simulink model "Project_Model"  (R2022b)
settings: Solver=ode45  StartTime=0.0  StopTime=1000  MaxStep=1  RelTol=1e-7
values from neighbouring files (symbols this model uses):
  a = (Rp+Ra)/2    [trial_complete_project.m]    (also in trial_detumbling.m; trial_earth_pointing.m)
  A0 = Ax*Ay*Az    [trial_complete_project.m]    (also in trial_detumbling.m = [0.5391 0.1008 0.8362; -0.3591 0.9255 0.1200; -0.7618 -0.365; trial_earth_pointing.m = [-0.2505 -0.7848 0.5668; 0.7978 0.1644 0.5801; -0.5485 0.597)
  A1 = L1*L2    (= 0.06)    [trial_complete_project.m]    (also in trial_detumbling.m; trial_earth_pointing.m)
  A10 = A1    (= 0.06)    [trial_complete_project.m]    (also in trial_detumbling.m; trial_earth_pointing.m)
  A2 = A1    (= 0.06)    [trial_complete_project.m]    (also in trial_detumbling.m; trial_earth_pointing.m)
  A3 = L1*L3    (= 0.03)    [trial_complete_project.m]    (also in trial_detumbling.m; trial_earth_pointing.m)
  A4 = A3    (= 0.03)    [trial_complete_project.m]    (also in trial_detumbling.m; trial_earth_pointing.m)
  A5 = L2*L3    (= 0.02)    [trial_complete_project.m]    (also in trial_detumbling.m; trial_earth_pointing.m)
  A6 = A5    (= 0.02)    [trial_complete_project.m]    (also in trial_detumbling.m; trial_earth_pointing.m)
  A7 = A1    (= 0.06)    [trial_complete_project.m]    (also in trial_detumbling.m; trial_earth_pointing.m)
  A8 = A1    (= 0.06)    [trial_complete_project.m]    (also in trial_detumbling.m; trial_earth_pointing.m)
  A9 = A1    (= 0.06)    [trial_complete_project.m]    (also in trial_detumbling.m; trial_earth_pointing.m)
  a_s = 149600000    [trial_complete_project.m]    (also in trial_detumbling.m; trial_earth_pointing.m)
  alpha1 = 0.9    [trial_complete_project.m]    (also in trial_detumbling.m; trial_earth_pointing.m)
  alpha2 = 0.1    [trial_complete_project.m]    (also in trial_detumbling.m; trial_earth_pointing.m)
  alphaState_obs = -0.9    [trial_complete_project.m]    (also in trial_detumbling.m; trial_earth_pointing.m)
  an = (11.5*pi)/180    (= 0.200712863979)    [trial_complete_project.m]    (also in trial_detumbling.m; trial_earth_pointing.m)
  d = 0.05/2    (= 0.025)    [trial_complete_project.m]    (also in trial_detumbling.m; trial_earth_pointing.m)
  e = (Ra-Rp)/(Ra+Rp)    [trial_complete_project.m]    (also in trial_detumbling.m; trial_earth_pointing.m)
  e_s = 0.0167086    [trial_complete_project.m]    (also in trial_detumbling.m; trial_earth_pointing.m)
  g_vect = g_vect'.*1e-9    [trial_complete_project.m]    (also in trial_detumbling.m; trial_earth_pointing.m)
  gamma = 30*pi/180    (= 0.523598775598)    [trial_complete_project.m]    (also in trial_detumbling.m; trial_earth_pointing.m)
  h_vect = h_vect'.*1e-9    [trial_complete_project.m]    (also in trial_detumbling.m; trial_earth_pointing.m)
  i = 0*pi/180    (= 0)    [trial_complete_project.m]    (also in trial_detumbling.m; trial_earth_pointing.m)
  I_x = 0.059029338    [trial_complete_project.m]    (also in trial_detumbling.m; trial_earth_pointing.m = 0.093296)
  I_y = 0.116709338    [trial_complete_project.m]    (also in trial_detumbling.m; trial_earth_pointing.m = 0.161261916)
  I_z = 0.149968    [trial_complete_project.m]    (also in trial_detumbling.m; trial_earth_pointing.m = 0.160253916)
  kdx = kd*(I_x/I)    (= 1.44987726319)    [trial_complete_project.m]    (also in trial_detumbling.m; trial_earth_pointing.m = 2.6989394073)
  kdy = kd*(I_y/I)    (= 2.86661211697)    [trial_complete_project.m]    (also in trial_detumbling.m; trial_earth_pointing.m = 4.66511040119)
  kdz = kd*(I_z/I)    (= 3.68351061984)    [trial_complete_project.m]    (also in trial_detumbling.m; trial_earth_pointing.m = 4.63595019151)
  kpx = kp*(I_x/I)    (= 0.0163111192108)    [trial_complete_project.m]    (also in trial_detumbling.m; trial_earth_pointing.m = 0.0202420455548)
  kpy = kp*(I_y/I)    (= 0.0322493863159)    [trial_complete_project.m]    (also in trial_detumbling.m; trial_earth_pointing.m = 0.0349883280089)
  kpz = kp*(I_z/I)    (= 0.0414394944732)    [trial_complete_project.m]    (also in trial_detumbling.m; trial_earth_pointing.m = 0.0347696264363)
  kState_obs = 0.9    [trial_complete_project.m]    (also in trial_detumbling.m; trial_earth_pointing.m)
  L = 0.3/2    (= 0.15)    [trial_complete_project.m]    (also in trial_detumbling.m; trial_earth_pointing.m)
  m = [0.01 0.05 0.01]    [trial_complete_project.m]    (also in trial_detumbling.m; trial_earth_pointing.m)
  MIB = 5*1e-3    (= 0.005)    [trial_complete_project.m]    (also in trial_detumbling.m; trial_earth_pointing.m)
  mu = astroConstants(13)    [trial_complete_project.m]    (also in trial_detumbling.m; trial_earth_pointing.m)
  n = sqrt(mu/a^3)    [trial_complete_project.m]    (also in trial_detumbling.m; trial_earth_pointing.m)
  n_B = 13    [trial_complete_project.m]    (also in trial_detumbling.m; trial_earth_pointing.m)
  n_s = sqrt(mu_s/a_s^3)    [trial_complete_project.m]    (also in trial_detumbling.m; trial_earth_pointing.m)
  P = F_e/c    (= 4.52980041279e-06)    [trial_complete_project.m]    (also in trial_detumbling.m; trial_earth_pointing.m)
  P_E = F_earth/c    (= 2.23487943783e-06)    [trial_complete_project.m]    (also in trial_detumbling.m; trial_earth_pointing.m)
  pd_sc = 0.1    [trial_complete_project.m]    (also in trial_detumbling.m; trial_earth_pointing.m)
  pd_sp = 0.1    [trial_complete_project.m]    (also in trial_detumbling.m; trial_earth_pointing.m)
  ps_sc = 0.5    [trial_complete_project.m]    (also in trial_detumbling.m; trial_earth_pointing.m)
  ps_sp = 0.1    [trial_complete_project.m]    (also in trial_detumbling.m; trial_earth_pointing.m)
  r = astroConstants(23)    [trial_complete_project.m]    (also in trial_detumbling.m; trial_earth_pointing.m)
  r1 = [0;0;-L3/2] + c_m    [trial_complete_project.m]    (also in trial_detumbling.m; trial_earth_pointing.m)
  r10 = r9    [trial_complete_project.m]    (also in trial_detumbling.m; trial_earth_pointing.m)
  r2 = [0; 0 ;L3/2] + c_m    [trial_complete_project.m]    (also in trial_detumbling.m; trial_earth_pointing.m)
  r3 = [0; L2/2;0] + c_m    [trial_complete_project.m]    (also in trial_detumbling.m; trial_earth_pointing.m)
  r4 = [0; -L2/2;0] + c_m    [trial_complete_project.m]    (also in trial_detumbling.m; trial_earth_pointing.m)
  r5 = [-L1/2; 0 ;0] + c_m    [trial_complete_project.m]    (also in trial_detumbling.m; trial_earth_pointing.m)
  r6 = [L1/2; 0;0]+ c_m    [trial_complete_project.m]    (also in trial_detumbling.m; trial_earth_pointing.m)
  r7 = [-L1/2; 0 ; L3/2 + L1/2] + c_m    [trial_complete_project.m]    (also in trial_detumbling.m; trial_earth_pointing.m)
  r8 = r7    [trial_complete_project.m]    (also in trial_detumbling.m; trial_earth_pointing.m)
  r9 = [-L1/2; 0 ; -L3/2 - L1/2]    [trial_complete_project.m]    (also in trial_detumbling.m; trial_earth_pointing.m)
  RW = 0.002    [trial_complete_project.m]    (also in trial_detumbling.m; trial_earth_pointing.m)
  theta0 = 0    [trial_complete_project.m]    (also in trial_detumbling.m; trial_earth_pointing.m)
  Thruster_Power = 0.03    [trial_complete_project.m]    (also in trial_detumbling.m; trial_earth_pointing.m)
  w = [1 1 1 1]'    [trial_complete_project.m]    (also in trial_detumbling.m; trial_earth_pointing.m)
  w0_x = 1    [trial_complete_project.m]    (also in trial_detumbling.m; trial_earth_pointing.m = -0.008328)
  w0_y = 1    [trial_complete_project.m]    (also in trial_detumbling.m; trial_earth_pointing.m = 0.004962)
  w0_z = 1    [trial_complete_project.m]    (also in trial_detumbling.m; trial_earth_pointing.m = -0.0004756)
  w_E = (15.04*pi/180)/3600    (= 7.29159776389e-05)    [trial_complete_project.m]    (also in trial_detumbling.m; trial_earth_pointing.m)
libraries: matrix_library x28, vrlib x6, dspinverses x2
(part 3 of 3)

== system Project_Model/Environment/Magnetic Torque/MAGNETIC FIELD ==
  S/C position : Inport
  Clock : Clock
  Constant1 : Constant  Value=g_vect
  Constant2 : Constant  Value=h_vect
  MATLAB Function1 : MATLAB Function  TreatAsAtomicUnit=on
  MATLAB Function2 : MATLAB Function  TreatAsAtomicUnit=on
  "order n " : Constant  Value=n_B
  B_n : Outport
  wires:
  Constant2/1 -> MATLAB Function1/7(hS)
  Constant1/1 -> MATLAB Function1/6(gS)
  MATLAB Function2/3(lat) -> MATLAB Function1/4(lat)
  MATLAB Function2/4(lon) -> MATLAB Function1/5(lon)
  Clock/1 -> MATLAB Function2/2(t)
  MATLAB Function2/1(r) -> MATLAB Function1/2(r)
  S/C position/1 -> MATLAB Function2/1(R)
  MATLAB Function2/2(alpha) -> MATLAB Function1/3(alpha)
  "order n "/1 -> MATLAB Function1/1(n_B)
  MATLAB Function1/1(B) -> B_n/1  "B_n"

== system Project_Model/Environment/Magnetic Torque/Theta_integration ==
  Constant : Constant
  Constant1 : Constant  Value=e
  Constant2 : Constant  Value=e
  Constant3 : Constant
  Constant4 : Constant  Value=3/2
  Cos : Trigonometry  Operator=cos
  Divide : Product  Inputs=*/
  Gain : Gain  Gain=n
  Integrator : Integrator  InitialCondition=theta0
  Product : Product
  Scope : Scope
  Scope1 : Scope
  Square : Math  Operator=square
  Square1 : Math  Operator=square
  Square2 : Math  Operator=pow
  Sum : Sum  Inputs=|++
  Sum1 : Sum  Inputs=|+-
  Output : Outport
  wires:
  Constant1/1 -> Product/1
  Integrator/1 -> Output/1, Scope/1, Cos/1
  Constant3/1 -> Sum1/1
  Cos/1 -> Product/2
  Product/1 -> Sum/1
  Square1/1 -> Sum1/2
  Constant/1 -> Sum/2
  Sum1/1 -> Square2/1
  Constant2/1 -> Square1/1
  Square/1 -> Gain/1
  Divide/1 -> Scope1/1, Integrator/1
  Sum/1 -> Square/1
  Square2/1 -> Divide/2
  Constant4/1 -> Square2/2
  Gain/1 -> Divide/1

== system Project_Model/Environment/Magnetic Torque/r_N ==
  Input1 : Inport
  Constant : Constant  Value=i
  Constant2 : Constant
  Constant3 : Constant  Value=e
  Constant4 : Constant
  Constant5 : Constant  Value=e
  Cos : Trigonometry  Operator=cos
  Cos1 : Trigonometry  Operator=cos
  Cos4 : Trigonometry  Operator=cos
  Divide : Product  Inputs=*/  RndMeth=Zero  SaturateOnIntegerOverflow=on
  Gain : Gain  Gain=a
  Product{,1,4..5} (4 alike) : Product
  Sin : Trigonometry
  Sin1 : Trigonometry
  Square : Math  Operator=square
  Sum : Sum  Inputs=|+-
  Sum1 : Sum  Inputs=|++
  Vector Concatenate : Concatenate  NumInputs=3
  Output : Outport
  wires:
  Input1/1 -> Cos4/1, Cos/1, Sin/1
  Constant/1 -> Sin1/1, Cos1/1
  Cos/1 -> Vector Concatenate/1
  Sin/1 -> Product1/1, Product/1
  Cos1/1 -> Product/2
  Product/1 -> Vector Concatenate/2
  Sin1/1 -> Product1/2
  Product1/1 -> Vector Concatenate/3
  Constant4/1 -> Sum1/1
  Product5/1 -> Output/1
  Constant2/1 -> Sum/1
  Cos4/1 -> Product4/2
  Sum1/1 -> Divide/2
  Constant3/1 -> Square/1
  Product4/1 -> Sum1/2
  Square/1 -> Sum/2
  Gain/1 -> Divide/1
  Sum/1 -> Gain/1
  Constant5/1 -> Product4/1
  Divide/1 -> Product5/1
  Vector Concatenate/1 -> Product5/2

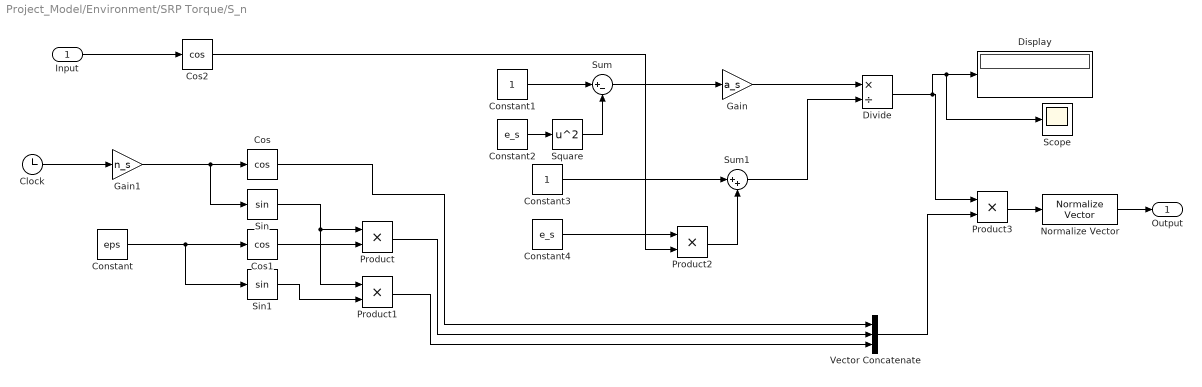
== system Project_Model/Environment/SRP Torque/S_n ==
  Input : Inport
  Clock : Clock
  Constant : Constant  Value=eps
  Constant1 : Constant
  Constant2 : Constant  Value=e_s
  Constant3 : Constant
  Constant4 : Constant  Value=e_s
  Cos : Trigonometry  Operator=cos
  Cos1 : Trigonometry  Operator=cos
  Cos2 : Trigonometry  Operator=cos
  Display : Display
  Divide : Product  Inputs=*/  RndMeth=Zero  SaturateOnIntegerOverflow=on
  Gain : Gain  Gain=a_s
  Gain1 : Gain  Gain=n_s
  Normalize Vector : vrlib/Utilities/Normalize Vector  maxzero=0
  Product{,1..3} (4 alike) : Product
  Scope : Scope
  Sin : Trigonometry
  Sin1 : Trigonometry
  Square : Math  Operator=square
  Sum : Sum  Inputs=|+-
  Sum1 : Sum  Inputs=|++
  Vector Concatenate : Concatenate  NumInputs=3
  Output : Outport
  wires:
  Product3/1 -> Normalize Vector/1
  Divide/1 -> Scope/1, Display/1, Product3/1
  Sum1/1 -> Divide/2
  Product2/1 -> Sum1/2
  Constant4/1 -> Product2/1
  Constant3/1 -> Sum1/1
  Gain/1 -> Divide/1
  Sum/1 -> Gain/1
  Square/1 -> Sum/2
  Constant2/1 -> Square/1
  Constant1/1 -> Sum/1
  Product1/1 -> Vector Concatenate/3
  Cos1/1 -> Product/2
  Sin1/1 -> Product1/2
  Constant/1 -> Cos1/1, Sin1/1
  Product/1 -> Vector Concatenate/2
  Cos/1 -> Vector Concatenate/1
  Sin/1 -> Product/1, Product1/1
  Vector Concatenate/1 -> Product3/2
  Clock/1 -> Gain1/1
  Gain1/1 -> Sin/1, Cos/1
  Input/1 -> Cos2/1
  Cos2/1 -> Product2/2
  Normalize Vector/1 -> Output/1

== system Project_Model/Environment/SRP Torque/Spacecraft Geometry ==
  Constant : Constant
  Gain : Gain  Gain=-1
  Gain1 : Gain  Gain=-1
  Gain2 : Gain  Gain=-1
  Vector Concatenate : Concatenate  NumInputs=3
  Vector Concatenate1 : Concatenate  NumInputs=3
  Vector Concatenate2 : Concatenate  NumInputs=3
  Zero : Constant  Value=0  OutDataTypeStr=Inherit: Inherit via back propagation
  Output : Outport
  Output1 : Outport  Port=2
  Output2 : Outport  Port=3
  Output3 : Outport  Port=4
  Output4 : Outport  Port=5
  Output5 : Outport  Port=6
  Output6 : Outport  Port=7
  Output7 : Outport  Port=8
  Output8 : Outport  Port=9
  Output9 : Outport  Port=10
  wires:
  Constant/1 -> Vector Concatenate2/3, Vector Concatenate/1, Vector Concatenate1/2
  Vector Concatenate1/1 -> Output3/1, Gain1/1
  Zero/1 -> Vector Concatenate2/2, Vector Concatenate2/1, Vector Concatenate1/3, Vector Concatenate/3, Vector Concatenate/2, Vector Concatenate1/1
  Vector Concatenate/1 -> Output8/1, Output6/1, Output4/1, Gain/1
  Vector Concatenate2/1 -> Gain2/1, Output/1
  Gain2/1 -> Output1/1
  Gain1/1 -> Output2/1
  Gain/1 -> Output9/1, Output7/1, Output5/1

== system Project_Model/Environment/SRP Torque/Subsystem ==
  Input : Inport
  Input1 : Inport  Port=2
  Constant : Constant
  Constant1 : Constant  Value=ps_sc
  Constant2 : Constant  Value=pd_sc
  Display : Display
  Dot Product : DotProduct  OutDataTypeStr=Inherit: Inherit via internal rule
  Gain : Gain  Gain=-P
  Gain1 : Gain  Gain=A1
  Gain2 : Gain  Gain=2
  Gain3 : Gain  Gain=2/3
  Product{,1..3} (4 alike) : Product
  Sum : Sum  Inputs=|+-
  Sum1 : Sum  Inputs=|++
  Sum2 : Sum  Inputs=|++
  Output : Outport
  Output1 : Outport  Port=2
  wires:
  Input1/1 -> Dot Product/2, Product3/2  "N_B"
  Product2/1 -> Sum2/1
  Product1/1 -> Sum1/1
  Constant2/1 -> Gain3/1
  Sum/1 -> Product1/1
  Constant1/1 -> Gain2/1, Sum/2
  Sum1/1 -> Product/2
  Product/1 -> Display/1, Output/1
  Dot Product/1 -> Output1/1, Product2/2, Gain/1
  Gain/1 -> Gain1/1
  Gain1/1 -> Product/1
  Sum2/1 -> Product3/1
  Input/1 -> Product1/2, Dot Product/1  "S-B"
  Gain2/1 -> Product2/1
  Constant/1 -> Sum/1
  Product3/1 -> Sum1/2
  Gain3/1 -> Sum2/2

== system Project_Model/Environment/SRP Torque/Subsystem10 ==
  Input : Inport
  Input1 : Inport  Port=2
  Constant : Constant
  Constant1 : Constant  Value=ps_sp
  Constant2 : Constant  Value=pd_sp
  Dot Product : DotProduct  OutDataTypeStr=Inherit: Inherit via internal rule
  Gain : Gain  Gain=-P
  Gain1 : Gain  Gain=A10
  Gain2 : Gain  Gain=2
  Gain3 : Gain  Gain=2/3
  Product{,1..3} (4 alike) : Product
  Sum : Sum  Inputs=|+-
  Sum1 : Sum  Inputs=|++
  Sum2 : Sum  Inputs=|++
  Output : Outport
  Output1 : Outport  Port=2
  wires:
  Gain3/1 -> Sum2/2
  Product3/1 -> Sum1/2
  Constant/1 -> Sum/1
  Gain2/1 -> Product2/1
  Input/1 -> Dot Product/1, Product1/2  "S-B"
  Sum2/1 -> Product3/1
  Gain1/1 -> Product/1
  Gain/1 -> Gain1/1
  Dot Product/1 -> Gain/1, Product2/2, Output1/1
  Product/1 -> Output/1
  Sum1/1 -> Product/2
  Constant1/1 -> Sum/2, Gain2/1
  Sum/1 -> Product1/1
  Constant2/1 -> Gain3/1
  Product1/1 -> Sum1/1
  Product2/1 -> Sum2/1
  Input1/1 -> Product3/2, Dot Product/2  "N_B"

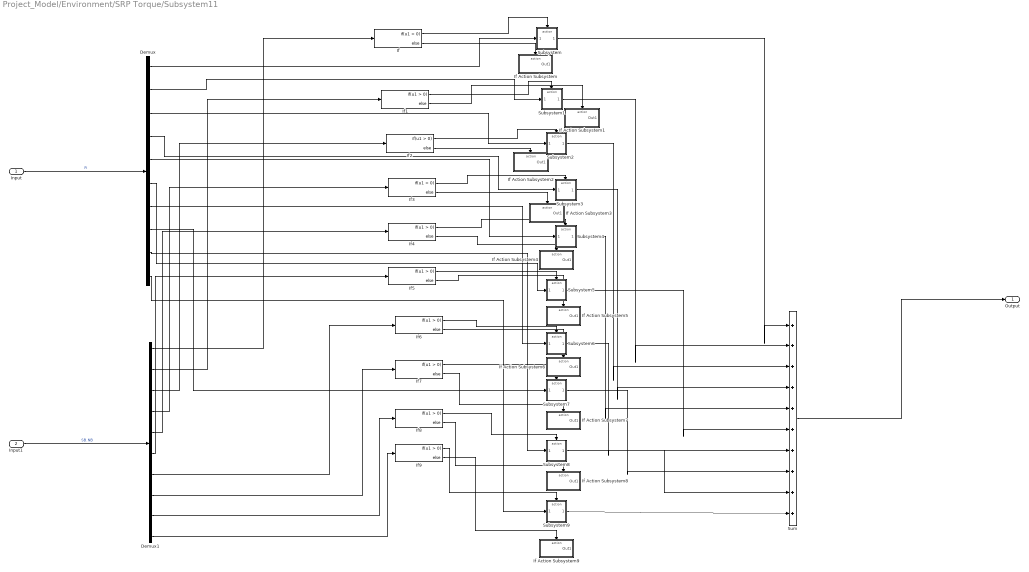
== system Project_Model/Environment/SRP Torque/Subsystem11 ==
  Input : Inport
  Input1 : Inport  Port=2
  Demux : Demux  Outputs=10
  Demux1 : Demux  Outputs=10
  If{,1..9} (10 alike) : If  ZeroCross=off
  If Action Subsystem : Subsystem  TreatAsAtomicUnit=on
  If Action Subsystem1 : Subsystem  TreatAsAtomicUnit=on
  If Action Subsystem2 : Subsystem  TreatAsAtomicUnit=on
  If Action Subsystem3 : Subsystem  TreatAsAtomicUnit=on
  If Action Subsystem4 : Subsystem  TreatAsAtomicUnit=on
  If Action Subsystem5 : Subsystem  TreatAsAtomicUnit=on
  If Action Subsystem6 : Subsystem  TreatAsAtomicUnit=on
  If Action Subsystem7 : Subsystem  TreatAsAtomicUnit=on
  If Action Subsystem8 : Subsystem  TreatAsAtomicUnit=on
  If Action Subsystem9 : Subsystem  TreatAsAtomicUnit=on
  Subsystem : Subsystem
  Subsystem1 : Subsystem
  Subsystem2 : Subsystem
  Subsystem3 : Subsystem
  Subsystem4 : Subsystem
  Subsystem5 : Subsystem
  Subsystem6 : Subsystem
  Subsystem7 : Subsystem
  Subsystem8 : Subsystem
  Subsystem9 : Subsystem
  Sum : Sum  Inputs=|++++++++++
  Output : Outport
  wires:
  Input/1 -> Demux/1  "Fi"
  Input1/1 -> Demux1/1  "SB.NB"
  Demux1/1 -> If/1
  Demux/1 -> Subsystem/1(Input3)
  Demux1/2 -> If1/1
  Demux1/3 -> If2/1
  Demux1/4 -> If3/1
  Demux1/5 -> If4/1
  Demux1/6 -> If5/1
  Demux1/7 -> If6/1
  Demux1/8 -> If7/1
  Demux1/9 -> If8/1
  Demux1/10 -> If9/1
  Demux/2 -> Subsystem1/1(Input3)
  Demux/3 -> Subsystem2/1(Input3)
  Demux/4 -> Subsystem3/1(Input3)
  Demux/5 -> Subsystem4/1(Input3)
  Demux/6 -> Subsystem5/1(Input3)
  Demux/7 -> Subsystem6/1(Input3)
  Demux/8 -> Subsystem7/1(Input3)
  Demux/9 -> Subsystem8/1(Input3)
  Demux/10 -> Subsystem9/1(Input3)
  Subsystem/1(Output) -> Sum/1
  Subsystem1/1(Output) -> Sum/2
  Subsystem2/1(Output) -> Sum/3
  Subsystem3/1(Output) -> Sum/4
  Subsystem4/1(Output) -> Sum/5
  Subsystem5/1(Output) -> Sum/6
  Subsystem6/1(Output) -> Sum/7
  Subsystem7/1(Output) -> Sum/8
  Subsystem8/1(Output) -> Sum/9
  Subsystem9/1(Output) -> Sum/10
  If/1 -> Subsystem/Action
  If/2 -> If Action Subsystem/Action
  If1/1 -> Subsystem1/Action
  If1/2 -> If Action Subsystem1/Action
  If2/2 -> If Action Subsystem2/Action
  If2/1 -> Subsystem2/Action
  If3/2 -> If Action Subsystem3/Action
  If3/1 -> Subsystem3/Action
  If4/2 -> If Action Subsystem4/Action
  If4/1 -> Subsystem4/Action
  If5/2 -> If Action Subsystem5/Action
  If5/1 -> Subsystem5/Action
  If6/2 -> If Action Subsystem6/Action
  If6/1 -> Subsystem6/Action
  If7/2 -> If Action Subsystem7/Action
  If7/1 -> Subsystem7/Action
  If8/2 -> If Action Subsystem8/Action
  If8/1 -> Subsystem8/Action
  If9/2 -> If Action Subsystem9/Action
  If9/1 -> Subsystem9/Action
  Sum/1 -> Output/1

== system Project_Model/Environment/SRP Torque/Subsystem2 ==
  Input : Inport
  Input1 : Inport  Port=2
  Constant : Constant
  Constant1 : Constant  Value=ps_sc
  Constant2 : Constant  Value=pd_sc
  Dot Product : DotProduct  OutDataTypeStr=Inherit: Inherit via internal rule
  Gain : Gain  Gain=-P
  Gain1 : Gain  Gain=A2
  Gain2 : Gain  Gain=2
  Gain3 : Gain  Gain=2/3
  Product{,1..3} (4 alike) : Product
  Sum : Sum  Inputs=|+-
  Sum1 : Sum  Inputs=|++
  Sum2 : Sum  Inputs=|++
  Output : Outport
  Output1 : Outport  Port=2
  wires:
  Gain3/1 -> Sum2/2
  Product3/1 -> Sum1/2
  Constant/1 -> Sum/1
  Gain2/1 -> Product2/1
  Input/1 -> Dot Product/1, Product1/2  "S-B"
  Sum2/1 -> Product3/1
  Gain1/1 -> Product/1
  Gain/1 -> Gain1/1
  Dot Product/1 -> Gain/1, Product2/2, Output1/1
  Product/1 -> Output/1
  Sum1/1 -> Product/2
  Constant1/1 -> Sum/2, Gain2/1
  Sum/1 -> Product1/1
  Constant2/1 -> Gain3/1
  Product1/1 -> Sum1/1
  Product2/1 -> Sum2/1
  Input1/1 -> Product3/2, Dot Product/2  "N_B"

== system Project_Model/Environment/SRP Torque/Subsystem3 ==
  Input : Inport
  Input1 : Inport  Port=2
  Constant : Constant
  Constant1 : Constant  Value=ps_sc
  Constant2 : Constant  Value=pd_sc
  Dot Product : DotProduct  OutDataTypeStr=Inherit: Inherit via internal rule
  Gain : Gain  Gain=-P
  Gain1 : Gain  Gain=A3
  Gain2 : Gain  Gain=2
  Gain3 : Gain  Gain=2/3
  Product{,1..3} (4 alike) : Product
  Sum : Sum  Inputs=|+-
  Sum1 : Sum  Inputs=|++
  Sum2 : Sum  Inputs=|++
  Output : Outport
  Output1 : Outport  Port=2
  wires:
  Input1/1 -> Dot Product/2, Product3/2  "N_B"
  Product2/1 -> Sum2/1
  Product1/1 -> Sum1/1
  Constant2/1 -> Gain3/1
  Sum/1 -> Product1/1
  Constant1/1 -> Gain2/1, Sum/2
  Sum1/1 -> Product/2
  Product/1 -> Output/1
  Dot Product/1 -> Output1/1, Product2/2, Gain/1
  Gain/1 -> Gain1/1
  Gain1/1 -> Product/1
  Sum2/1 -> Product3/1
  Input/1 -> Product1/2, Dot Product/1  "S-B"
  Gain2/1 -> Product2/1
  Constant/1 -> Sum/1
  Product3/1 -> Sum1/2
  Gain3/1 -> Sum2/2

== system Project_Model/Environment/SRP Torque/Subsystem4 ==
  Input : Inport
  Input1 : Inport  Port=2
  Constant : Constant
  Constant1 : Constant  Value=ps_sc
  Constant2 : Constant  Value=pd_sc
  Dot Product : DotProduct  OutDataTypeStr=Inherit: Inherit via internal rule
  Gain : Gain  Gain=-P
  Gain1 : Gain  Gain=A4
  Gain2 : Gain  Gain=2
  Gain3 : Gain  Gain=2/3
  Product{,1..3} (4 alike) : Product
  Sum : Sum  Inputs=|+-
  Sum1 : Sum  Inputs=|++
  Sum2 : Sum  Inputs=|++
  Output : Outport
  Output1 : Outport  Port=2
  wires:
  Gain3/1 -> Sum2/2
  Product3/1 -> Sum1/2
  Constant/1 -> Sum/1
  Gain2/1 -> Product2/1
  Input/1 -> Dot Product/1, Product1/2  "S-B"
  Sum2/1 -> Product3/1
  Gain1/1 -> Product/1
  Gain/1 -> Gain1/1
  Dot Product/1 -> Gain/1, Product2/2, Output1/1
  Product/1 -> Output/1
  Sum1/1 -> Product/2
  Constant1/1 -> Sum/2, Gain2/1
  Sum/1 -> Product1/1
  Constant2/1 -> Gain3/1
  Product1/1 -> Sum1/1
  Product2/1 -> Sum2/1
  Input1/1 -> Product3/2, Dot Product/2  "N_B"

== system Project_Model/Environment/SRP Torque/Subsystem5 ==
  Input : Inport
  Input1 : Inport  Port=2
  Constant : Constant
  Constant1 : Constant  Value=ps_sc
  Constant2 : Constant  Value=pd_sc
  Dot Product : DotProduct  OutDataTypeStr=Inherit: Inherit via internal rule
  Gain : Gain  Gain=-P
  Gain1 : Gain  Gain=A5
  Gain2 : Gain  Gain=2
  Gain3 : Gain  Gain=2/3
  Product{,1..3} (4 alike) : Product
  Sum : Sum  Inputs=|+-
  Sum1 : Sum  Inputs=|++
  Sum2 : Sum  Inputs=|++
  Output : Outport
  Output1 : Outport  Port=2
  wires:
  Input1/1 -> Dot Product/2, Product3/2  "N_B"
  Product2/1 -> Sum2/1
  Product1/1 -> Sum1/1
  Constant2/1 -> Gain3/1
  Sum/1 -> Product1/1
  Constant1/1 -> Gain2/1, Sum/2
  Sum1/1 -> Product/2
  Product/1 -> Output/1
  Dot Product/1 -> Output1/1, Product2/2, Gain/1
  Gain/1 -> Gain1/1
  Gain1/1 -> Product/1
  Sum2/1 -> Product3/1
  Input/1 -> Product1/2, Dot Product/1  "S-B"
  Gain2/1 -> Product2/1
  Constant/1 -> Sum/1
  Product3/1 -> Sum1/2
  Gain3/1 -> Sum2/2

== system Project_Model/Environment/SRP Torque/Subsystem6 ==
  Input : Inport
  Input1 : Inport  Port=2
  Constant : Constant
  Constant1 : Constant  Value=ps_sc
  Constant2 : Constant  Value=pd_sc
  Dot Product : DotProduct  OutDataTypeStr=Inherit: Inherit via internal rule
  Gain : Gain  Gain=-P
  Gain1 : Gain  Gain=A6
  Gain2 : Gain  Gain=2
  Gain3 : Gain  Gain=2/3
  Product{,1..3} (4 alike) : Product
  Sum : Sum  Inputs=|+-
  Sum1 : Sum  Inputs=|++
  Sum2 : Sum  Inputs=|++
  Output : Outport
  Output1 : Outport  Port=2
  wires:
  Gain3/1 -> Sum2/2
  Product3/1 -> Sum1/2
  Constant/1 -> Sum/1
  Gain2/1 -> Product2/1
  Input/1 -> Dot Product/1, Product1/2  "S-B"
  Sum2/1 -> Product3/1
  Gain1/1 -> Product/1
  Gain/1 -> Gain1/1
  Dot Product/1 -> Gain/1, Product2/2, Output1/1
  Product/1 -> Output/1
  Sum1/1 -> Product/2
  Constant1/1 -> Sum/2, Gain2/1
  Sum/1 -> Product1/1
  Constant2/1 -> Gain3/1
  Product1/1 -> Sum1/1
  Product2/1 -> Sum2/1
  Input1/1 -> Product3/2, Dot Product/2  "N_B"

== system Project_Model/Environment/SRP Torque/Subsystem7 ==
  Input : Inport
  Input1 : Inport  Port=2
  Constant : Constant
  Constant1 : Constant  Value=ps_sp
  Constant2 : Constant  Value=pd_sp
  Dot Product : DotProduct  OutDataTypeStr=Inherit: Inherit via internal rule
  Gain : Gain  Gain=-P
  Gain1 : Gain  Gain=A7
  Gain2 : Gain  Gain=2
  Gain3 : Gain  Gain=2/3
  Product{,1..3} (4 alike) : Product
  Sum : Sum  Inputs=|+-
  Sum1 : Sum  Inputs=|++
  Sum2 : Sum  Inputs=|++
  Output : Outport
  Output1 : Outport  Port=2
  wires:
  Input1/1 -> Dot Product/2, Product3/2  "N_B"
  Product2/1 -> Sum2/1
  Product1/1 -> Sum1/1
  Constant2/1 -> Gain3/1
  Sum/1 -> Product1/1
  Constant1/1 -> Gain2/1, Sum/2
  Sum1/1 -> Product/2
  Product/1 -> Output/1
  Dot Product/1 -> Output1/1, Product2/2, Gain/1
  Gain/1 -> Gain1/1
  Gain1/1 -> Product/1
  Sum2/1 -> Product3/1
  Input/1 -> Product1/2, Dot Product/1  "S-B"
  Gain2/1 -> Product2/1
  Constant/1 -> Sum/1
  Product3/1 -> Sum1/2
  Gain3/1 -> Sum2/2

== system Project_Model/Environment/SRP Torque/Subsystem8 ==
  Input : Inport
  Input1 : Inport  Port=2
  Constant : Constant
  Constant1 : Constant  Value=ps_sp
  Constant2 : Constant  Value=pd_sp
  Dot Product : DotProduct  OutDataTypeStr=Inherit: Inherit via internal rule
  Gain : Gain  Gain=-P
  Gain1 : Gain  Gain=A8
  Gain2 : Gain  Gain=2
  Gain3 : Gain  Gain=2/3
  Product{,1..3} (4 alike) : Product
  Sum : Sum  Inputs=|+-
  Sum1 : Sum  Inputs=|++
  Sum2 : Sum  Inputs=|++
  Output : Outport
  Output1 : Outport  Port=2
  wires:
  Gain3/1 -> Sum2/2
  Product3/1 -> Sum1/2
  Constant/1 -> Sum/1
  Gain2/1 -> Product2/1
  Input/1 -> Dot Product/1, Product1/2  "S-B"
  Sum2/1 -> Product3/1
  Gain1/1 -> Product/1
  Gain/1 -> Gain1/1
  Dot Product/1 -> Gain/1, Product2/2, Output1/1
  Product/1 -> Output/1
  Sum1/1 -> Product/2
  Constant1/1 -> Sum/2, Gain2/1
  Sum/1 -> Product1/1
  Constant2/1 -> Gain3/1
  Product1/1 -> Sum1/1
  Product2/1 -> Sum2/1
  Input1/1 -> Product3/2, Dot Product/2  "N_B"

== system Project_Model/Environment/SRP Torque/Subsystem9 ==
  Input : Inport
  Input1 : Inport  Port=2
  Constant : Constant
  Constant1 : Constant  Value=ps_sp
  Constant2 : Constant  Value=pd_sp
  Dot Product : DotProduct  OutDataTypeStr=Inherit: Inherit via internal rule
  Gain : Gain  Gain=-P
  Gain1 : Gain  Gain=A9
  Gain2 : Gain  Gain=2
  Gain3 : Gain  Gain=2/3
  Product{,1..3} (4 alike) : Product
  Sum : Sum  Inputs=|+-
  Sum1 : Sum  Inputs=|++
  Sum2 : Sum  Inputs=|++
  Output : Outport
  Output1 : Outport  Port=2
  wires:
  Input1/1 -> Dot Product/2, Product3/2  "N_B"
  Product2/1 -> Sum2/1
  Product1/1 -> Sum1/1
  Constant2/1 -> Gain3/1
  Sum/1 -> Product1/1
  Constant1/1 -> Gain2/1, Sum/2
  Sum1/1 -> Product/2
  Product/1 -> Output/1
  Dot Product/1 -> Output1/1, Product2/2, Gain/1
  Gain/1 -> Gain1/1
  Gain1/1 -> Product/1
  Sum2/1 -> Product3/1
  Input/1 -> Product1/2, Dot Product/1  "S-B"
  Gain2/1 -> Product2/1
  Constant/1 -> Sum/1
  Product3/1 -> Sum1/2
  Gain3/1 -> Sum2/2

== system Project_Model/Environment/SRP Torque/Theta_integration ==
  Constant : Constant
  Constant1 : Constant  Value=e
  Constant2 : Constant  Value=e
  Constant3 : Constant
  Constant4 : Constant  Value=3/2
  Cos : Trigonometry  Operator=cos
  Divide : Product  Inputs=*/
  Gain : Gain  Gain=n
  Integrator : Integrator  InitialCondition=theta0
  Product : Product
  Scope : Scope
  Square : Math  Operator=square
  Square1 : Math  Operator=square
  Square2 : Math  Operator=pow
  Sum : Sum  Inputs=|++
  Sum1 : Sum  Inputs=|+-
  Output : Outport
  wires:
  Gain/1 -> Divide/1
  Constant4/1 -> Square2/2
  Square2/1 -> Divide/2
  Sum/1 -> Square/1
  Divide/1 -> Integrator/1
  Square/1 -> Gain/1
  Constant2/1 -> Square1/1
  Sum1/1 -> Square2/1
  Constant/1 -> Sum/2
  Square1/1 -> Sum1/2
  Product/1 -> Sum/1
  Cos/1 -> Product/2
  Constant3/1 -> Sum1/1
  Integrator/1 -> Cos/1, Scope/1, Output/1
  Constant1/1 -> Product/1

== system Project_Model/Reaction Wheel/If Action Subsystem/If Action Subsystem ==
  Action Port : ActionPort  ActionPortLabel=if(u1 <RWmin)
  Constant : Constant  Value=0
  Out1 : Outport
  wires:
  Constant/1 -> Out1/1

== system Project_Model/Reaction Wheel/If Action Subsystem/If Action Subsystem1 ==
  Action Port : ActionPort  ActionPortLabel=elseif(u1>=RW)
  Constant : Constant  Value=RW
  Out1 : Outport
  wires:
  Constant/1 -> Out1/1

== system Project_Model/Reaction Wheel/If Action Subsystem/If Action Subsystem2 ==
  Input : Inport
  Action Port : ActionPort  ActionPortLabel=else
  Out1 : Outport
  wires:
  Input/1 -> Out1/1

== system Project_Model/Reaction Wheel/If Action Subsystem1/If Action Subsystem ==
  Action Port : ActionPort  ActionPortLabel=if(u1 >-RWmin)
  Constant : Constant  Value=0
  Out1 : Outport
  wires:
  Constant/1 -> Out1/1

== system Project_Model/Reaction Wheel/If Action Subsystem1/If Action Subsystem1 ==
  Action Port : ActionPort  ActionPortLabel=elseif(u1<=-RW)
  Constant : Constant  Value=-RW
  Out1 : Outport
  wires:
  Constant/1 -> Out1/1

== system Project_Model/Reaction Wheel/If Action Subsystem1/If Action Subsystem2 ==
  Input : Inport
  Action Port : ActionPort  ActionPortLabel=else
  Out1 : Outport
  wires:
  Input/1 -> Out1/1

== system Project_Model/Reaction Wheel/If Action Subsystem2/If Action Subsystem ==
  Action Port : ActionPort  ActionPortLabel=if(u1 <RWmin)
  Constant : Constant  Value=0
  Out1 : Outport
  wires:
  Constant/1 -> Out1/1

== system Project_Model/Reaction Wheel/If Action Subsystem2/If Action Subsystem1 ==
  Action Port : ActionPort  ActionPortLabel=elseif(u1>=RW)
  Constant : Constant  Value=RW
  Out1 : Outport
  wires:
  Constant/1 -> Out1/1

== system Project_Model/Reaction Wheel/If Action Subsystem2/If Action Subsystem2 ==
  Input : Inport
  Action Port : ActionPort  ActionPortLabel=else
  Out1 : Outport
  wires:
  Input/1 -> Out1/1

== system Project_Model/Reaction Wheel/If Action Subsystem3/If Action Subsystem ==
  Action Port : ActionPort  ActionPortLabel=if(u1 >-RWmin)
  Constant : Constant  Value=0
  Out1 : Outport
  wires:
  Constant/1 -> Out1/1

== system Project_Model/Reaction Wheel/If Action Subsystem3/If Action Subsystem1 ==
  Action Port : ActionPort  ActionPortLabel=elseif(u1<=-RW)
  Constant : Constant  Value=-RW
  Out1 : Outport
  wires:
  Constant/1 -> Out1/1

== system Project_Model/Reaction Wheel/If Action Subsystem3/If Action Subsystem2 ==
  Input : Inport
  Action Port : ActionPort  ActionPortLabel=else
  Out1 : Outport
  wires:
  Input/1 -> Out1/1

== system Project_Model/Reaction Wheel/If Action Subsystem4/If Action Subsystem ==
  Action Port : ActionPort  ActionPortLabel=if(u1 <RWmin)
  Constant : Constant  Value=0
  Out1 : Outport
  wires:
  Constant/1 -> Out1/1

== system Project_Model/Reaction Wheel/If Action Subsystem4/If Action Subsystem1 ==
  Action Port : ActionPort  ActionPortLabel=elseif(u1>=RW)
  Constant : Constant  Value=RW
  Out1 : Outport
  wires:
  Constant/1 -> Out1/1

== system Project_Model/Reaction Wheel/If Action Subsystem4/If Action Subsystem2 ==
  Input : Inport
  Action Port : ActionPort  ActionPortLabel=else
  Out1 : Outport
  wires:
  Input/1 -> Out1/1

== system Project_Model/Reaction Wheel/If Action Subsystem5/If Action Subsystem ==
  Action Port : ActionPort  ActionPortLabel=if(u1 >-RWmin)
  Constant : Constant  Value=0
  Out1 : Outport
  wires:
  Constant/1 -> Out1/1

== system Project_Model/Reaction Wheel/If Action Subsystem5/If Action Subsystem1 ==
  Action Port : ActionPort  ActionPortLabel=elseif(u1<=-RW)
  Constant : Constant  Value=-RW
  Out1 : Outport
  wires:
  Constant/1 -> Out1/1

== system Project_Model/Reaction Wheel/If Action Subsystem5/If Action Subsystem2 ==
  Input : Inport
  Action Port : ActionPort  ActionPortLabel=else
  Out1 : Outport
  wires:
  Input/1 -> Out1/1

== system Project_Model/Environment/ERP Torque/Subsystem11/If Action Subsystem ==
  Action Port : ActionPort  ActionPortLabel=else
  Constant : Constant  Value=[0 0 0]'
  Out1 : Outport
  wires:
  Constant/1 -> Out1/1

== system Project_Model/Environment/ERP Torque/Subsystem11/If Action Subsystem1 ==
  Action Port : ActionPort  ActionPortLabel=else
  Constant : Constant  Value=[0 0 0]'
  Out1 : Outport
  wires:
  Constant/1 -> Out1/1

== system Project_Model/Environment/ERP Torque/Subsystem11/If Action Subsystem2 ==
  Action Port : ActionPort  ActionPortLabel=else
  Constant : Constant  Value=[0 0 0]'
  Out1 : Outport
  wires:
  Constant/1 -> Out1/1

== system Project_Model/Environment/ERP Torque/Subsystem11/If Action Subsystem3 ==
  Action Port : ActionPort  ActionPortLabel=else
  Constant : Constant  Value=[0 0 0]'
  Out1 : Outport
  wires:
  Constant/1 -> Out1/1

== system Project_Model/Environment/ERP Torque/Subsystem11/If Action Subsystem4 ==
  Action Port : ActionPort  ActionPortLabel=else
  Constant : Constant  Value=[0 0 0]'
  Out1 : Outport
  wires:
  Constant/1 -> Out1/1

== system Project_Model/Environment/ERP Torque/Subsystem11/If Action Subsystem5 ==
  Action Port : ActionPort  ActionPortLabel=else
  Constant : Constant  Value=[0 0 0]'
  Out1 : Outport
  wires:
  Constant/1 -> Out1/1

== system Project_Model/Environment/ERP Torque/Subsystem11/If Action Subsystem6 ==
  Action Port : ActionPort  ActionPortLabel=else
  Constant : Constant  Value=[0 0 0]'
  Out1 : Outport
  wires:
  Constant/1 -> Out1/1

== system Project_Model/Environment/ERP Torque/Subsystem11/If Action Subsystem7 ==
  Action Port : ActionPort  ActionPortLabel=else
  Constant : Constant  Value=[0 0 0]'
  Out1 : Outport
  wires:
  Constant/1 -> Out1/1

== system Project_Model/Environment/ERP Torque/Subsystem11/If Action Subsystem8 ==
  Action Port : ActionPort  ActionPortLabel=else
  Constant : Constant  Value=[0 0 0]'
  Out1 : Outport
  wires:
  Constant/1 -> Out1/1

== system Project_Model/Environment/ERP Torque/Subsystem11/If Action Subsystem9 ==
  Action Port : ActionPort  ActionPortLabel=else
  Constant : Constant  Value=[0 0 0]'
  Out1 : Outport
  wires:
  Constant/1 -> Out1/1

== system Project_Model/Environment/ERP Torque/Subsystem11/Subsystem ==
  Input3 : Inport
  Action Port : ActionPort  ActionPortLabel=if(u1 > 0)
  Constant : Constant  Value=r1
  Cross Product : matrix_library/Cross Product
  Output : Outport
  wires:
  Cross Product/1 -> Output/1
  Constant/1 -> Cross Product/1
  Input3/1 -> Cross Product/2

== system Project_Model/Environment/ERP Torque/Subsystem11/Subsystem1 ==
  Input3 : Inport
  Action Port : ActionPort  ActionPortLabel=if(u1 > 0)
  Constant : Constant  Value=r2
  Cross Product : matrix_library/Cross Product
  Output : Outport
  wires:
  Input3/1 -> Cross Product/2
  Constant/1 -> Cross Product/1
  Cross Product/1 -> Output/1

== system Project_Model/Environment/ERP Torque/Subsystem11/Subsystem2 ==
  Input3 : Inport
  Action Port : ActionPort  ActionPortLabel=if(u1 > 0)
  Constant : Constant  Value=r3
  Cross Product : matrix_library/Cross Product
  Output : Outport
  wires:
  Cross Product/1 -> Output/1
  Constant/1 -> Cross Product/1
  Input3/1 -> Cross Product/2

== system Project_Model/Environment/ERP Torque/Subsystem11/Subsystem3 ==
  Input3 : Inport
  Action Port : ActionPort  ActionPortLabel=if(u1 > 0)
  Constant : Constant  Value=r4
  Cross Product : matrix_library/Cross Product
  Output : Outport
  wires:
  Input3/1 -> Cross Product/2
  Constant/1 -> Cross Product/1
  Cross Product/1 -> Output/1

== system Project_Model/Environment/ERP Torque/Subsystem11/Subsystem4 ==
  Input3 : Inport
  Action Port : ActionPort  ActionPortLabel=if(u1 > 0)
  Constant : Constant  Value=r5
  Cross Product : matrix_library/Cross Product
  Output : Outport
  wires:
  Cross Product/1 -> Output/1
  Constant/1 -> Cross Product/1
  Input3/1 -> Cross Product/2

== system Project_Model/Environment/ERP Torque/Subsystem11/Subsystem5 ==
  Input3 : Inport
  Action Port : ActionPort  ActionPortLabel=if(u1 > 0)
  Constant : Constant  Value=r6
  Cross Product : matrix_library/Cross Product
  Output : Outport
  wires:
  Input3/1 -> Cross Product/2
  Constant/1 -> Cross Product/1
  Cross Product/1 -> Output/1

== system Project_Model/Environment/ERP Torque/Subsystem11/Subsystem6 ==
  Input3 : Inport
  Action Port : ActionPort  ActionPortLabel=if(u1 > 0)
  Constant : Constant  Value=r7
  Cross Product : matrix_library/Cross Product
  Output : Outport
  wires:
  Cross Product/1 -> Output/1
  Constant/1 -> Cross Product/1
  Input3/1 -> Cross Product/2

== system Project_Model/Environment/ERP Torque/Subsystem11/Subsystem7 ==
  Input3 : Inport
  Action Port : ActionPort  ActionPortLabel=if(u1 > 0)
  Constant : Constant  Value=r8
  Cross Product : matrix_library/Cross Product
  Output : Outport
  wires:
  Input3/1 -> Cross Product/2
  Constant/1 -> Cross Product/1
  Cross Product/1 -> Output/1

== system Project_Model/Environment/ERP Torque/Subsystem11/Subsystem8 ==
  Input3 : Inport
  Action Port : ActionPort  ActionPortLabel=if(u1 > 0)
  Constant : Constant  Value=r9
  Cross Product : matrix_library/Cross Product
  Display : Display
  Output : Outport
  wires:
  Cross Product/1 -> Output/1
  Constant/1 -> Cross Product/1
  Input3/1 -> Cross Product/2, Display/1

== system Project_Model/Environment/ERP Torque/Subsystem11/Subsystem9 ==
  Input3 : Inport
  Action Port : ActionPort  ActionPortLabel=if(u1 > 0)
  Constant : Constant  Value=r10
  Cross Product : matrix_library/Cross Product
  Output : Outport
  wires:
  Input3/1 -> Cross Product/2
  Constant/1 -> Cross Product/1
  Cross Product/1 -> Output/1

== system Project_Model/Environment/Gravity Torque/Two_body_problem/R ==
  Input : Inport
  Constant1 : Constant
  Constant2 : Constant  Value=e
  Constant3 : Constant
  Constant4 : Constant  Value=e
  Cos2 : Trigonometry  Operator=cos
  Divide : Product  Inputs=*/  RndMeth=Zero  SaturateOnIntegerOverflow=on
  Gain : Gain  Gain=a
  Product2 : Product
  Square : Math  Operator=square
  Sum : Sum  Inputs=|+-
  Sum1 : Sum  Inputs=|++
  Output : Outport
  wires:
  Sum1/1 -> Divide/2
  Product2/1 -> Sum1/2
  Constant4/1 -> Product2/1
  Constant3/1 -> Sum1/1
  Gain/1 -> Divide/1
  Sum/1 -> Gain/1
  Square/1 -> Sum/2
  Constant2/1 -> Square/1
  Constant1/1 -> Sum/1
  Input/1 -> Cos2/1
  Cos2/1 -> Product2/2
  Divide/1 -> Output/1

== system Project_Model/Environment/Gravity Torque/Two_body_problem/Theta_integration ==
  Constant : Constant
  Constant1 : Constant  Value=e
  Constant2 : Constant  Value=e
  Constant3 : Constant
  Constant4 : Constant  Value=3/2
  Cos : Trigonometry  Operator=cos
  Divide : Product  Inputs=*/
  Gain : Gain  Gain=n
  Integrator : Integrator  InitialCondition=theta0
  Product : Product
  Scope : Scope
  Square : Math  Operator=square
  Square1 : Math  Operator=square
  Square2 : Math  Operator=pow
  Sum : Sum  Inputs=|++
  Sum1 : Sum  Inputs=|+-
  Output : Outport
  wires:
  Constant1/1 -> Product/1
  Integrator/1 -> Output/1, Scope/1, Cos/1
  Constant3/1 -> Sum1/1
  Cos/1 -> Product/2
  Product/1 -> Sum/1
  Square1/1 -> Sum1/2
  Constant/1 -> Sum/2
  Sum1/1 -> Square2/1
  Constant2/1 -> Square1/1
  Square/1 -> Gain/1
  Divide/1 -> Integrator/1
  Sum/1 -> Square/1
  Square2/1 -> Divide/2
  Constant4/1 -> Square2/2
  Gain/1 -> Divide/1

== system Project_Model/Environment/SRP Torque/Subsystem11/If Action Subsystem ==
  Action Port : ActionPort  ActionPortLabel=else
  Constant : Constant  Value=[0 0 0]'
  Out1 : Outport
  wires:
  Constant/1 -> Out1/1

== system Project_Model/Environment/SRP Torque/Subsystem11/If Action Subsystem1 ==
  Action Port : ActionPort  ActionPortLabel=else
  Constant : Constant  Value=[0 0 0]'
  Out1 : Outport
  wires:
  Constant/1 -> Out1/1

== system Project_Model/Environment/SRP Torque/Subsystem11/If Action Subsystem2 ==
  Action Port : ActionPort  ActionPortLabel=else
  Constant : Constant  Value=[0 0 0]'
  Out1 : Outport
  wires:
  Constant/1 -> Out1/1

== system Project_Model/Environment/SRP Torque/Subsystem11/If Action Subsystem3 ==
  Action Port : ActionPort  ActionPortLabel=else
  Constant : Constant  Value=[0 0 0]'
  Out1 : Outport
  wires:
  Constant/1 -> Out1/1

== system Project_Model/Environment/SRP Torque/Subsystem11/If Action Subsystem4 ==
  Action Port : ActionPort  ActionPortLabel=else
  Constant : Constant  Value=[0 0 0]'
  Out1 : Outport
  wires:
  Constant/1 -> Out1/1

== system Project_Model/Environment/SRP Torque/Subsystem11/If Action Subsystem5 ==
  Action Port : ActionPort  ActionPortLabel=else
  Constant : Constant  Value=[0 0 0]'
  Out1 : Outport
  wires:
  Constant/1 -> Out1/1

== system Project_Model/Environment/SRP Torque/Subsystem11/If Action Subsystem6 ==
  Action Port : ActionPort  ActionPortLabel=else
  Constant : Constant  Value=[0 0 0]'
  Out1 : Outport
  wires:
  Constant/1 -> Out1/1

== system Project_Model/Environment/SRP Torque/Subsystem11/If Action Subsystem7 ==
  Action Port : ActionPort  ActionPortLabel=else
  Constant : Constant  Value=[0 0 0]'
  Out1 : Outport
  wires:
  Constant/1 -> Out1/1

== system Project_Model/Environment/SRP Torque/Subsystem11/If Action Subsystem8 ==
  Action Port : ActionPort  ActionPortLabel=else
  Constant : Constant  Value=[0 0 0]'
  Out1 : Outport
  wires:
  Constant/1 -> Out1/1

== system Project_Model/Environment/SRP Torque/Subsystem11/If Action Subsystem9 ==
  Action Port : ActionPort  ActionPortLabel=else
  Constant : Constant  Value=[0 0 0]'
  Out1 : Outport
  wires:
  Constant/1 -> Out1/1

== system Project_Model/Environment/SRP Torque/Subsystem11/Subsystem ==
  Input3 : Inport
  Action Port : ActionPort  ActionPortLabel=if(u1 > 0)
  Constant : Constant  Value=r1
  Cross Product : matrix_library/Cross Product
  Output : Outport
  wires:
  Input3/1 -> Cross Product/2
  Constant/1 -> Cross Product/1
  Cross Product/1 -> Output/1

== system Project_Model/Environment/SRP Torque/Subsystem11/Subsystem1 ==
  Input3 : Inport
  Action Port : ActionPort  ActionPortLabel=if(u1 > 0)
  Constant : Constant  Value=r2
  Cross Product : matrix_library/Cross Product
  Output : Outport
  wires:
  Cross Product/1 -> Output/1
  Constant/1 -> Cross Product/1
  Input3/1 -> Cross Product/2

== system Project_Model/Environment/SRP Torque/Subsystem11/Subsystem2 ==
  Input3 : Inport
  Action Port : ActionPort  ActionPortLabel=if(u1 > 0)
  Constant : Constant  Value=r3
  Cross Product : matrix_library/Cross Product
  Output : Outport
  wires:
  Input3/1 -> Cross Product/2
  Constant/1 -> Cross Product/1
  Cross Product/1 -> Output/1

== system Project_Model/Environment/SRP Torque/Subsystem11/Subsystem3 ==
  Input3 : Inport
  Action Port : ActionPort  ActionPortLabel=if(u1 > 0)
  Constant : Constant  Value=r4
  Cross Product : matrix_library/Cross Product
  Output : Outport
  wires:
  Cross Product/1 -> Output/1
  Constant/1 -> Cross Product/1
  Input3/1 -> Cross Product/2

== system Project_Model/Environment/SRP Torque/Subsystem11/Subsystem4 ==
  Input3 : Inport
  Action Port : ActionPort  ActionPortLabel=if(u1 > 0)
  Constant : Constant  Value=r5
  Cross Product : matrix_library/Cross Product
  Output : Outport
  wires:
  Input3/1 -> Cross Product/2
  Constant/1 -> Cross Product/1
  Cross Product/1 -> Output/1

== system Project_Model/Environment/SRP Torque/Subsystem11/Subsystem5 ==
  Input3 : Inport
  Action Port : ActionPort  ActionPortLabel=if(u1 > 0)
  Constant : Constant  Value=r6
  Cross Product : matrix_library/Cross Product
  Output : Outport
  wires:
  Cross Product/1 -> Output/1
  Constant/1 -> Cross Product/1
  Input3/1 -> Cross Product/2

== system Project_Model/Environment/SRP Torque/Subsystem11/Subsystem6 ==
  Input3 : Inport
  Action Port : ActionPort  ActionPortLabel=if(u1 > 0)
  Constant : Constant  Value=r7
  Cross Product : matrix_library/Cross Product
  Output : Outport
  wires:
  Input3/1 -> Cross Product/2
  Constant/1 -> Cross Product/1
  Cross Product/1 -> Output/1

== system Project_Model/Environment/SRP Torque/Subsystem11/Subsystem7 ==
  Input3 : Inport
  Action Port : ActionPort  ActionPortLabel=if(u1 > 0)
  Constant : Constant  Value=r8
  Cross Product : matrix_library/Cross Product
  Output : Outport
  wires:
  Cross Product/1 -> Output/1
  Constant/1 -> Cross Product/1
  Input3/1 -> Cross Product/2

== system Project_Model/Environment/SRP Torque/Subsystem11/Subsystem8 ==
  Input3 : Inport
  Action Port : ActionPort  ActionPortLabel=if(u1 > 0)
  Constant : Constant  Value=r9
  Cross Product : matrix_library/Cross Product
  Display : Display
  Output : Outport
  wires:
  Input3/1 -> Display/1, Cross Product/2
  Constant/1 -> Cross Product/1
  Cross Product/1 -> Output/1

== system Project_Model/Environment/SRP Torque/Subsystem11/Subsystem9 ==
  Input3 : Inport
  Action Port : ActionPort  ActionPortLabel=if(u1 > 0)
  Constant : Constant  Value=r10
  Cross Product : matrix_library/Cross Product
  Output : Outport
  wires:
  Cross Product/1 -> Output/1
  Constant/1 -> Cross Product/1
  Input3/1 -> Cross Product/2

== matlab function Project_Model/Attitude Determination/MATLAB Function ==
  data: B input; U output; M output; V output
function [U,M,V]  = fcn(B)

[U,S,V] = svd(B);

M=diag([1 1 det(U)*det(V)]);

end

== matlab function Project_Model/Environment/Magnetic Torque/MAGNETIC FIELD/MATLAB Function1 ==
  data: n_B input; B output; r input; alpha input; lat input; lon input; gS input; hS input
function B = magn_field (n_B, r, alpha, lat, lon, gS, hS)
%Function that models Earth magnetic field.

%Earth reference radius value used in IGRF
a=6371.2; 

%Colatitude
th=pi/2-lat;
%East longitude from Greenwich:
phi=lon;

%Variables definition:
    sum_br=0;
    sum_bth=0;
    sum_bphi=0;
    Br=0;
    Bth=0;
    Bphi=0;
    
    %Matrices:
    P=zeros (n_B+1); %Matrix of Gaussian normalized associated Legendre polynomials
    dP_th=zeros (n_B+1); %Matrix of derivatives of P wrt th

% Recursive computation of Lagrange polynomials:
    P(1,1)=1;
    dP_th(1,1)=0;

    i=1; 

    for n=1:n_B
        for m=0:n

            if m==n
                P(n+1,m+1)= sin(th)*P(n,n);
                dP_th(n+1,m+1)= sin(th)*dP_th(n,n) + cos(th)*P(n,n);
            else
                K = ((n-1)^2-m^2)/((2*n-1)*(2*n-3));
                if n==1
                    P(n+1,m+1)= cos(th)*P(n,m+1);
                    dP_th(n+1,m+1)= cos(th)*dP_th(n,m+1) - sin(th)*P(n,m+1);
                else 
                    P(n+1,m+1)= cos(th)*P(n,m+1)-K*P(n-1,m+1);
                    dP_th(n+1,m+1)= cos(th)*dP_th(n,m+1) - sin(th)*P(n,m+1) - ...
                        K*dP_th(n-1,m+1);
                end
            end
        
        gnm=gS(i);
        hnm=hS(i);
        
        sum_br= sum_br + (gnm*cos(m*phi) + hnm*sin(m*phi)) * P(n+1,m+1);
        sum_bth= sum_bth + (gnm*cos(m*phi) + hnm*sin(m*phi)) * dP_th(n+1,m+1);
        sum_bphi= sum_bphi + m*(-gnm*sin(m*phi) + hnm*cos(m*phi)) * P(n+1,m+1);
        
        i=i+1;
        
    end

%B vector components in (r,th,phi) frame:

   Br=Br+ ((a/r)^(n+2)) * (n+1) * sum_br;
   Bth=Bth+ (a/r)^(n+2) * sum_bth;
   Bphi=Bphi+ (a/r)^(n+2) * sum_bphi;
   
end

Bth= -Bth; 
Bphi= -Bphi/sin(th);

% Coordinate transformation: (r,th,phi)-> ECI frame
Bx= (Br*cos(lat) +Bth*sin(lat))*cos(alpha)-Bphi*sin(alpha);
By= (Br*cos(lat) +Bth*sin(lat))* sin(alpha) + Bphi*cos(alpha);
Bz= Br*sin(lat)- Bth*cos(lat);

%B vector:
B=[Bx; By; Bz];

== matlab function Project_Model/Environment/Magnetic Torque/MAGNETIC FIELD/MATLAB Function2 ==
  data: r output; R input; alpha output; lat output; lon output; t input
function [r,alpha,lat,lon]= input_definitions (R,t)

%Initial true anomaly at Greenwich Meridian:
theta_g_0=0;
%Earth Angular velocity @ its spin axis:
omega_E=15.04*2*pi/360/3600;


x=R(1); %x-coordinates of the S/C on the orbit
y=R(2); %y-coordinates of the S/C on the orbit
z=R(3); %z-coordinates of the S/C on the orbit

% Declination:
    r= sqrt(x^2+y^2+z^2); %norm of the position vector
    delta=asin( z/r ); %vector of angles [242x1]
% Right Ascension:
        if (y/r)>0
            alpha=acos( x/(r*cos(delta)) );
        else
            alpha=2*pi-acos( x/(r*cos(delta)) );
        end

theta_g=theta_g_0+omega_E*(t);
%Longitude:
    lon=alpha-theta_g;
%Latitude:
    lat=delta;
end
